simulink model "my_sim"  (R2023b)
settings: Solver=VariableStepAuto  StartTime=0.0  StopTime=2  FixedStep=0.001  MaxStep=0.001  RelTol=1e-3
values from neighbouring files (symbols this model uses):
  Bm = 0.02    [denklemler.m]    (also in my_params.m)
  Freq = 50    [my_params.m]
  J = 0.030    (= 0.03)    [denklemler.m]    (also in my_params.m)
  L1lr = 0.012    [denklemler.m]    (also in my_params.m)
  Lls = 0.008    [denklemler.m]    (also in my_params.m)
  Lm = 0.46    [denklemler.m]    (also in my_params.m)
  P = 2    [denklemler.m]    (also in my_params.m)
  R1r = 1.7    [my_params.m]
  Rs = 2    [denklemler.m]    (also in my_params.m)
  Vampl = 325    [my_params.m]
  w = 2*pi*Freq    (= 314.159265359)    [my_params.m]
libraries: simulink x2, spsabctodq0Lib x1
settings Model: Creator=enesb  LastModifiedBy=enesb
settings DataIOCC: ExternalInput=[inits]  SaveFormat=Array

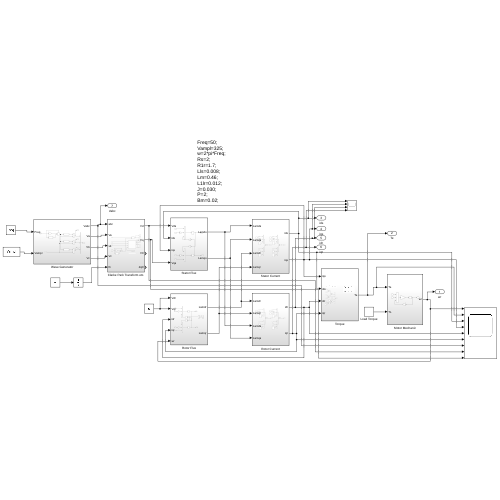
[thumbnail: Simulink's stored preview of the top-level diagram]
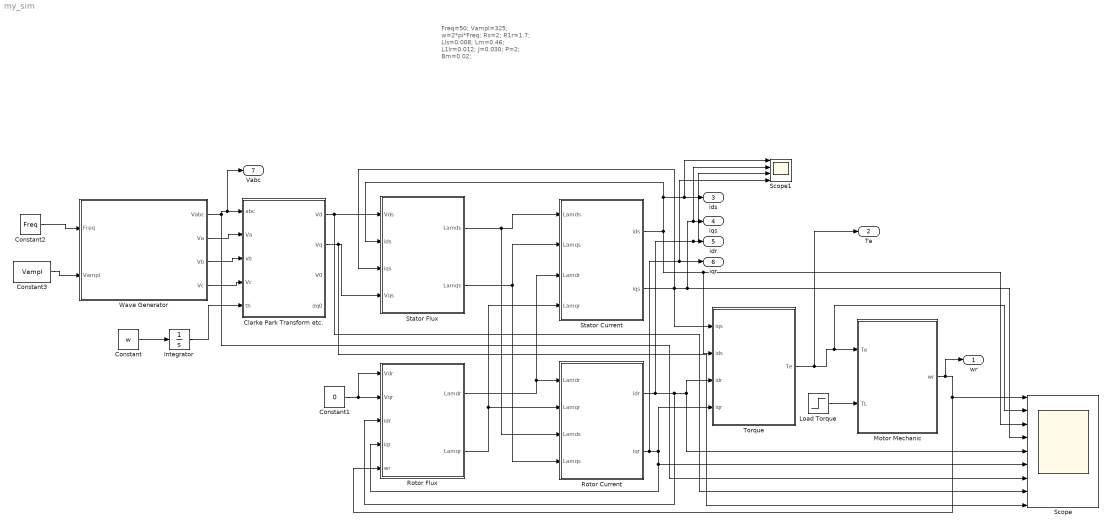
== system my_sim ==
  note: Freq=50;
      | Vampl=325;
      | w=2*pi*Freq;
      | Rs=2;
      | R1r=1.7;
      | Lls=0.008;
      | Lm=0.46;
      | L1lr=0.012;
      | J=0.030;
      | P=2;
      | Bm=0.02;
  Clarke Park Transform etc. : Subsystem
  Constant : Constant  Value=w
  Constant1 : Constant  Value=0
  Constant2 : Constant  Value=Freq
  Constant3 : Constant  Value=Vampl
  Integrator : Integrator
  Load Torque : Step  SampleTime=0
  Motor Mechanic : Subsystem
  Rotor Current : Subsystem
  Rotor Flux : Subsystem
  Scope : Scope  NumInputPorts=9
  Scope1 : Scope  NumInputPorts=4
  Stator Current : Subsystem
  Stator Flux : Subsystem
  Torque : Subsystem
  Wave Generator : Subsystem
  wr : Outport
  Te : Outport  Port=2
  ids : Outport  Port=3
  iqs : Outport  Port=4
  idr : Outport  Port=5
  iqr : Outport  Port=6
  Vabc : Outport  Port=7
  wires:
  Constant2/1 -> Wave Generator/1(Freq)
  Constant3/1 -> Wave Generator/2(Vampl)
  Constant/1 -> Integrator/1
  Wave Generator/1(Vabc) -> Vabc/1, Clarke Park Transform etc./1(abc), Scope/7
  Wave Generator/2(Va) -> Clarke Park Transform etc./2(Va)
  Wave Generator/3(Vb) -> Clarke Park Transform etc./3(vb)
  Wave Generator/4(Vc) -> Clarke Park Transform etc./4(Vc)
  Integrator/1 -> Clarke Park Transform etc./5(th)
  Clarke Park Transform etc./1(Vd) -> Scope/8, Stator Flux/1(Vds)
  Stator Current/1(ids) -> Scope/3, Torque/2(ids), Scope1/1, ids/1, Stator Flux/2(ids)
  Stator Flux/1(Lamds) -> Rotor Current/3(Lamds), Stator Current/1(Lamds)
  Stator Flux/2(Lamqs) -> Stator Current/2(Lamqs), Rotor Current/4(Lamqs)
  Rotor Flux/1(Lamdr) -> Rotor Current/1(Lamdr), Stator Current/3(Lamdr)
  Rotor Flux/2(Lamqr) -> Rotor Current/2(Lamqr), Stator Current/4(Lamqr)
  Clarke Park Transform etc./2(Vq) -> Scope/9, Stator Flux/4(Vqs)
  Rotor Current/1(idr) -> Scope1/3, idr/1, Scope/5, Torque/3(idr), Rotor Flux/3(idr)
  Rotor Current/2(iqr) -> iqr/1, Scope1/4, Torque/4(iqr), Scope/6, Rotor Flux/4(iqr)
  Motor Mechanic/1(wr) -> wr/1, Rotor Flux/5(wr), Scope/1
  Torque/1(Te) -> Te/1, Scope/2, Motor Mechanic/1(Te)
  Load Torque/1 -> Motor Mechanic/2(TL)
  Constant1/1 -> Rotor Flux/1(Vdr), Rotor Flux/2(Vqr)
  Stator Current/2(iqs) -> Scope1/2, iqs/1, Scope/4, Torque/1(iqs), Stator Flux/3(iqs)

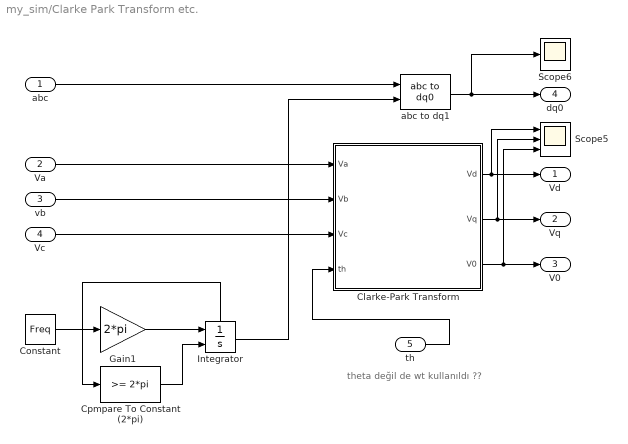
== system my_sim/Clarke Park Transform etc. ==
  note: theta değil de wt kullanıldı ??
  abc : Inport
  Va : Inport  Port=2
  vb : Inport  Port=3
  Vc : Inport  Port=4
  th : Inport  Port=5
  Clarke-Park Transform : MATLAB Function  TreatAsAtomicUnit=on
  Constant : Constant  Value=Freq
  Cpmpare To Constant (2*pi) : simulink/Logic and Bit Operations/Compare To Constant  relop=>=  const=2*pi  OutDataTypeStr=boolean
  Gain1 : Gain  Gain=2*pi
  Integrator : Integrator  ExternalReset=rising  ShowStatePort=on
  Scope5 : Scope  NumInputPorts=3
  Scope6 : Scope
  abc to dq1 : spsabctodq0Lib/abc to dq0  Alignment=90 degrees behind phase A axis
  Vd : Outport
  Vq : Outport  Port=2
  V0 : Outport  Port=3
  dq0 : Outport  Port=4
  wires:
  Vc/1 -> Clarke-Park Transform/3(Vc)
  vb/1 -> Clarke-Park Transform/2(Vb)
  Va/1 -> Clarke-Park Transform/1(Va)
  abc/1 -> abc to dq1/1
  Integrator/1 -> abc to dq1/2
  abc to dq1/1 -> Scope6/1, dq0/1
  Constant/1 -> Gain1/1
  Gain1/1 -> Integrator/1
  Cpmpare To Constant (2*pi)/1 -> Integrator/2
  Integrator/State -> Cpmpare To Constant (2*pi)/1
  Clarke-Park Transform/1(Vd) -> Scope5/1, Vd/1
  Clarke-Park Transform/2(Vq) -> Scope5/2, Vq/1
  Clarke-Park Transform/3(V0) -> Scope5/3, V0/1
  th/1 -> Clarke-Park Transform/4(th)

== system my_sim/Motor Mechanic ==
  Te : Inport
  TL : Inport  Port=2
  Add : Sum  Inputs=+--
  Gain : Gain  Gain=P/(2*J)
  Gain1 : Gain  Gain=Bm
  Integrator1 : Integrator
  wr : Outport
  wires:
  Add/1 -> Gain/1
  TL/1 -> Add/2
  Gain1/1 -> Add/3
  Gain/1 -> Integrator1/1
  Te/1 -> Add/1
  Integrator1/1 -> wr/1, Gain1/1

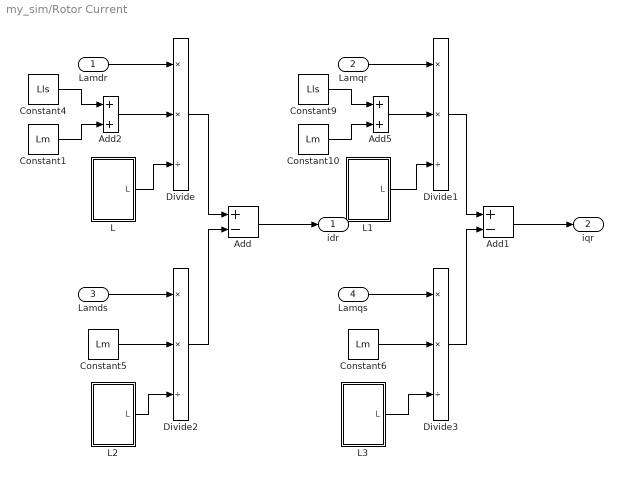
== system my_sim/Rotor Current ==
  Lamdr : Inport
  Lamqr : Inport  Port=2
  Lamds : Inport  Port=3
  Lamqs : Inport  Port=4
  Add : Sum  Inputs=+-
  Add1 : Sum  Inputs=+-
  Add2 : Sum
  Add5 : Sum
  Constant{1,5..6,10} (4 alike) : Constant  Value=Lm
  Constant4 : Constant  Value=Lls
  Constant9 : Constant  Value=Lls
  Divide{,1..3} (4 alike) : Product  Inputs=**/
  L : Subsystem
  L1 : Subsystem
  L2 : Subsystem
  L3 : Subsystem
  idr : Outport
  iqr : Outport  Port=2
  wires:
  Constant4/1 -> Add2/1
  L2/1(L) -> Divide2/3
  L3/1(L) -> Divide3/3
  Add2/1 -> Divide/2
  Constant9/1 -> Add5/1
  Constant1/1 -> Add2/2
  Divide1/1 -> Add1/1
  L1/1(L) -> Divide1/3
  Lamds/1 -> Divide2/1
  Divide3/1 -> Add1/2
  Constant10/1 -> Add5/2
  Add5/1 -> Divide1/2
  L/1(L) -> Divide/3
  Lamdr/1 -> Divide/1
  Constant5/1 -> Divide2/2
  Divide/1 -> Add/1
  Lamqr/1 -> Divide1/1
  Constant6/1 -> Divide3/2
  Lamqs/1 -> Divide3/1
  Add/1 -> idr/1
  Add1/1 -> iqr/1
  Divide2/1 -> Add/2

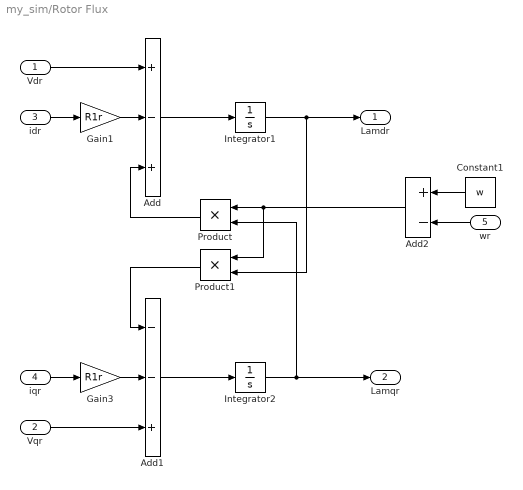
== system my_sim/Rotor Flux ==
  Vdr : Inport
  Vqr : Inport  Port=2
  idr : Inport  Port=3
  iqr : Inport  Port=4
  wr : Inport  Port=5
  Add : Sum  Inputs=+-+
  Add1 : Sum  Inputs=--+
  Add2 : Sum  Inputs=+-
  Constant1 : Constant  Value=w
  Gain1 : Gain  Gain=R1r
  Gain3 : Gain  Gain=R1r
  Integrator1 : Integrator
  Integrator2 : Integrator
  Product : Product
  Product1 : Product
  Lamdr : Outport
  Lamqr : Outport  Port=2
  wires:
  idr/1 -> Gain1/1
  Constant1/1 -> Add2/1
  Product/1 -> Add/3
  Vdr/1 -> Add/1
  Integrator2/1 -> Lamqr/1, Product/2
  iqr/1 -> Gain3/1
  Integrator1/1 -> Lamdr/1, Product1/2
  Gain1/1 -> Add/2
  Vqr/1 -> Add1/3
  Gain3/1 -> Add1/2
  Add/1 -> Integrator1/1
  Add1/1 -> Integrator2/1
  Product1/1 -> Add1/1
  Add2/1 -> Product1/1, Product/1
  wr/1 -> Add2/2

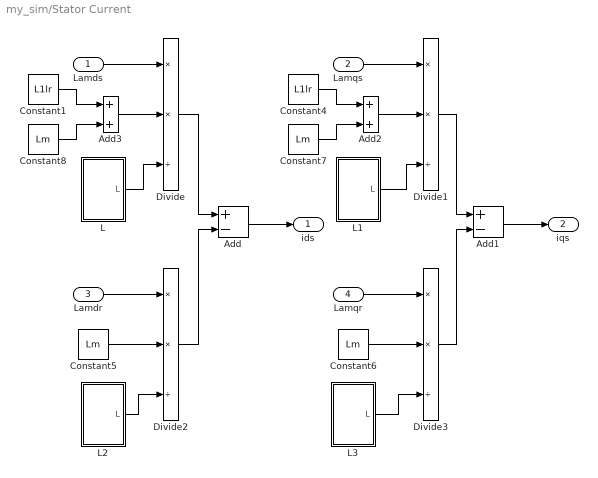
== system my_sim/Stator Current ==
  Lamds : Inport
  Lamqs : Inport  Port=2
  Lamdr : Inport  Port=3
  Lamqr : Inport  Port=4
  Add : Sum  Inputs=+-
  Add1 : Sum  Inputs=+-
  Add2 : Sum
  Add3 : Sum
  Constant1 : Constant  Value=L1lr
  Constant4 : Constant  Value=L1lr
  Constant{5..8} (4 alike) : Constant  Value=Lm
  Divide{,1..3} (4 alike) : Product  Inputs=**/
  L : Subsystem
  L1 : Subsystem
  L2 : Subsystem
  L3 : Subsystem
  ids : Outport
  iqs : Outport  Port=2
  wires:
  Lamqs/1 -> Divide1/1
  Add1/1 -> iqs/1
  Add3/1 -> Divide/2
  L1/1(L) -> Divide1/3
  Add2/1 -> Divide1/2
  Lamqr/1 -> Divide3/1
  Constant5/1 -> Divide2/2
  Lamds/1 -> Divide/1
  Divide1/1 -> Add1/1
  L/1(L) -> Divide/3
  Constant6/1 -> Divide3/2
  Constant8/1 -> Add3/2
  Constant7/1 -> Add2/2
  Constant4/1 -> Add2/1
  L3/1(L) -> Divide3/3
  Constant1/1 -> Add3/1
  Divide2/1 -> Add/2
  Divide/1 -> Add/1
  Lamdr/1 -> Divide2/1
  Divide3/1 -> Add1/2
  Add/1 -> ids/1
  L2/1(L) -> Divide2/3

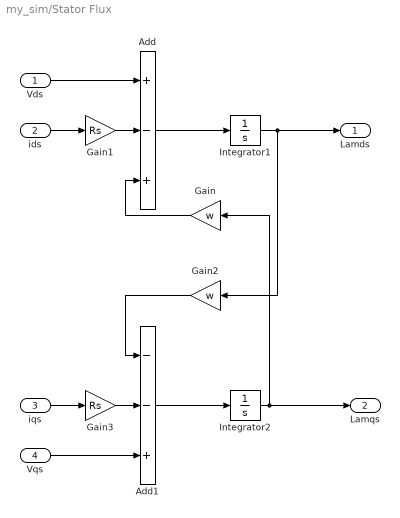
== system my_sim/Stator Flux ==
  Vds : Inport
  ids : Inport  Port=2
  iqs : Inport  Port=3
  Vqs : Inport  Port=4
  Add : Sum  Inputs=+-+
  Add1 : Sum  Inputs=--+
  Gain : Gain  Gain=w
  Gain1 : Gain  Gain=Rs
  Gain2 : Gain  Gain=w
  Gain3 : Gain  Gain=Rs
  Integrator1 : Integrator
  Integrator2 : Integrator
  Lamds : Outport
  Lamqs : Outport  Port=2
  wires:
  Gain1/1 -> Add/2
  ids/1 -> Gain1/1
  Vqs/1 -> Add1/3
  iqs/1 -> Gain3/1
  Gain2/1 -> Add1/1
  Gain/1 -> Add/3
  Vds/1 -> Add/1
  Gain3/1 -> Add1/2
  Integrator2/1 -> Lamqs/1, Gain/1
  Add/1 -> Integrator1/1
  Add1/1 -> Integrator2/1
  Integrator1/1 -> Lamds/1, Gain2/1

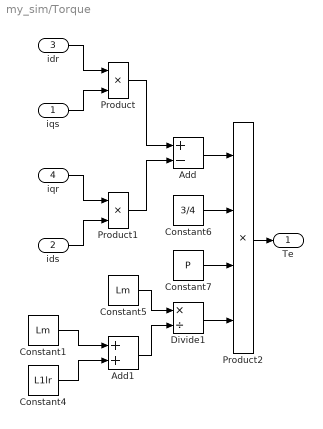
== system my_sim/Torque ==
  iqs : Inport
  ids : Inport  Port=2
  idr : Inport  Port=3
  iqr : Inport  Port=4
  Add : Sum  Inputs=+-
  Add1 : Sum
  Constant1 : Constant  Value=Lm
  Constant4 : Constant  Value=L1lr
  Constant5 : Constant  Value=Lm
  Constant6 : Constant  Value=3/4
  Constant7 : Constant  Value=P
  Divide1 : Product  Inputs=*/
  Product : Product
  Product1 : Product
  Product2 : Product  Inputs=4
  Te : Outport
  wires:
  iqr/1 -> Product1/1
  idr/1 -> Product/1
  Constant6/1 -> Product2/2
  Constant7/1 -> Product2/3
  Constant5/1 -> Divide1/1
  Add1/1 -> Divide1/2
  Product/1 -> Add/1
  Product1/1 -> Add/2
  Constant1/1 -> Add1/1
  iqs/1 -> Product/2
  Product2/1 -> Te/1
  ids/1 -> Product1/2
  Divide1/1 -> Product2/4
  Constant4/1 -> Add1/2
  Add/1 -> Product2/1

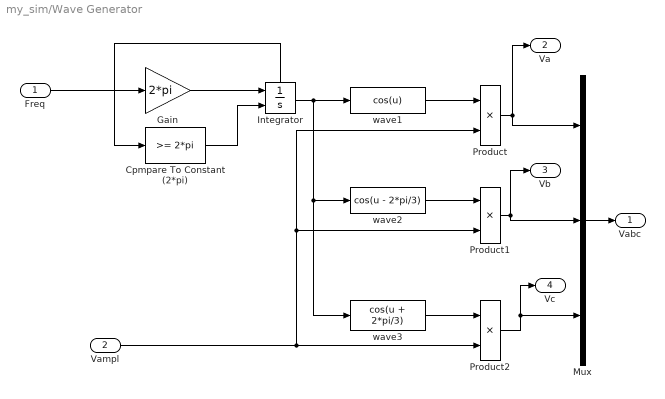
== system my_sim/Wave Generator ==
  Freq : Inport
  Vampl : Inport  Port=2
  Cpmpare To Constant (2*pi) : simulink/Logic and Bit Operations/Compare To Constant  relop=>=  const=2*pi  OutDataTypeStr=boolean
  Gain : Gain  Gain=2*pi
  Integrator : Integrator  ExternalReset=rising  ShowStatePort=on
  Mux : Mux  Inputs=3
  Product : Product
  Product1 : Product
  Product2 : Product
  wave1 : Fcn  Expr=cos(u)
  wave2 : Fcn  Expr=cos(u - 2*pi/3)
  wave3 : Fcn  Expr=cos(u + 2*pi/3)
  Vabc : Outport
  Va : Outport  Port=2
  Vb : Outport  Port=3
  Vc : Outport  Port=4
  wires:
  wave3/1 -> Product2/1
  Product/1 -> Va/1, Mux/1
  wave2/1 -> Product1/1
  Integrator/State -> Cpmpare To Constant (2*pi)/1
  Mux/1 -> Vabc/1
  Gain/1 -> Integrator/1
  Vampl/1 -> Product/2, Product1/2, Product2/2
  wave1/1 -> Product/1
  Cpmpare To Constant (2*pi)/1 -> Integrator/2
  Integrator/1 -> wave1/1, wave3/1, wave2/1
  Product2/1 -> Vc/1, Mux/3
  Product1/1 -> Vb/1, Mux/2
  Freq/1 -> Gain/1

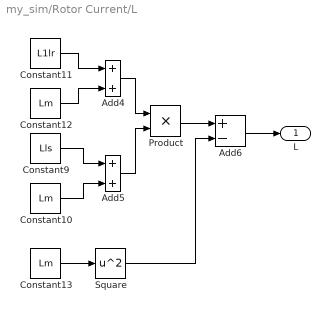
== system my_sim/Rotor Current/L ==
  Add4 : Sum
  Add5 : Sum
  Add6 : Sum  Inputs=+-
  Constant10 : Constant  Value=Lm
  Constant11 : Constant  Value=L1lr
  Constant12 : Constant  Value=Lm
  Constant13 : Constant  Value=Lm
  Constant9 : Constant  Value=Lls
  Product : Product
  Square : Math  Operator=square
  L : Outport
  wires:
  Product/1 -> Add6/1
  Constant12/1 -> Add4/2
  Constant10/1 -> Add5/2
  Add4/1 -> Product/1
  Constant11/1 -> Add4/1
  Constant9/1 -> Add5/1
  Add6/1 -> L/1
  Add5/1 -> Product/2
  Constant13/1 -> Square/1
  Square/1 -> Add6/2

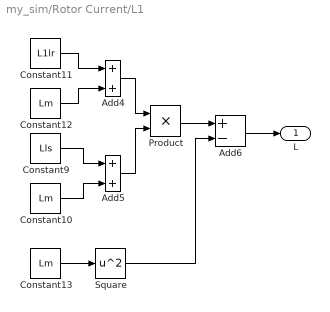
== system my_sim/Rotor Current/L1 ==
  Add4 : Sum
  Add5 : Sum
  Add6 : Sum  Inputs=+-
  Constant10 : Constant  Value=Lm
  Constant11 : Constant  Value=L1lr
  Constant12 : Constant  Value=Lm
  Constant13 : Constant  Value=Lm
  Constant9 : Constant  Value=Lls
  Product : Product
  Square : Math  Operator=square
  L : Outport
  wires:
  Square/1 -> Add6/2
  Constant13/1 -> Square/1
  Add5/1 -> Product/2
  Add6/1 -> L/1
  Constant9/1 -> Add5/1
  Constant11/1 -> Add4/1
  Add4/1 -> Product/1
  Constant10/1 -> Add5/2
  Constant12/1 -> Add4/2
  Product/1 -> Add6/1

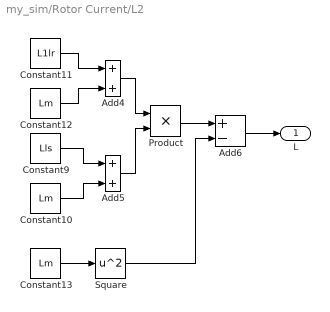
== system my_sim/Rotor Current/L2 ==
  Add4 : Sum
  Add5 : Sum
  Add6 : Sum  Inputs=+-
  Constant10 : Constant  Value=Lm
  Constant11 : Constant  Value=L1lr
  Constant12 : Constant  Value=Lm
  Constant13 : Constant  Value=Lm
  Constant9 : Constant  Value=Lls
  Product : Product
  Square : Math  Operator=square
  L : Outport
  wires:
  Square/1 -> Add6/2
  Constant13/1 -> Square/1
  Add5/1 -> Product/2
  Add6/1 -> L/1
  Constant9/1 -> Add5/1
  Constant11/1 -> Add4/1
  Add4/1 -> Product/1
  Constant10/1 -> Add5/2
  Constant12/1 -> Add4/2
  Product/1 -> Add6/1

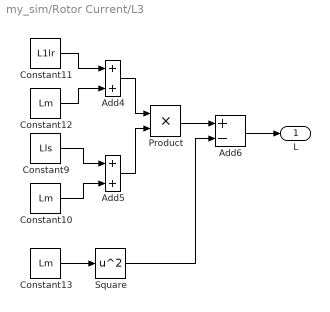
== system my_sim/Rotor Current/L3 ==
  Add4 : Sum
  Add5 : Sum
  Add6 : Sum  Inputs=+-
  Constant10 : Constant  Value=Lm
  Constant11 : Constant  Value=L1lr
  Constant12 : Constant  Value=Lm
  Constant13 : Constant  Value=Lm
  Constant9 : Constant  Value=Lls
  Product : Product
  Square : Math  Operator=square
  L : Outport
  wires:
  Product/1 -> Add6/1
  Constant12/1 -> Add4/2
  Constant10/1 -> Add5/2
  Add4/1 -> Product/1
  Constant11/1 -> Add4/1
  Constant9/1 -> Add5/1
  Add6/1 -> L/1
  Add5/1 -> Product/2
  Constant13/1 -> Square/1
  Square/1 -> Add6/2

== system my_sim/Stator Current/L ==
  Add4 : Sum
  Add5 : Sum
  Add6 : Sum  Inputs=+-
  Constant10 : Constant  Value=Lm
  Constant11 : Constant  Value=L1lr
  Constant12 : Constant  Value=Lm
  Constant13 : Constant  Value=Lm
  Constant9 : Constant  Value=Lls
  Product : Product
  Square : Math  Operator=square
  L : Outport
  wires:
  Product/1 -> Add6/1
  Constant12/1 -> Add4/2
  Constant10/1 -> Add5/2
  Add4/1 -> Product/1
  Constant11/1 -> Add4/1
  Constant9/1 -> Add5/1
  Add6/1 -> L/1
  Add5/1 -> Product/2
  Constant13/1 -> Square/1
  Square/1 -> Add6/2

== system my_sim/Stator Current/L1 ==
  Add4 : Sum
  Add5 : Sum
  Add6 : Sum  Inputs=+-
  Constant10 : Constant  Value=Lm
  Constant11 : Constant  Value=L1lr
  Constant12 : Constant  Value=Lm
  Constant13 : Constant  Value=Lm
  Constant9 : Constant  Value=Lls
  Product : Product
  Square : Math  Operator=square
  L : Outport
  wires:
  Square/1 -> Add6/2
  Constant13/1 -> Square/1
  Add5/1 -> Product/2
  Add6/1 -> L/1
  Constant9/1 -> Add5/1
  Constant11/1 -> Add4/1
  Add4/1 -> Product/1
  Constant10/1 -> Add5/2
  Constant12/1 -> Add4/2
  Product/1 -> Add6/1

== system my_sim/Stator Current/L2 ==
  Add4 : Sum
  Add5 : Sum
  Add6 : Sum  Inputs=+-
  Constant10 : Constant  Value=Lm
  Constant11 : Constant  Value=L1lr
  Constant12 : Constant  Value=Lm
  Constant13 : Constant  Value=Lm
  Constant9 : Constant  Value=Lls
  Product : Product
  Square : Math  Operator=square
  L : Outport
  wires:
  Square/1 -> Add6/2
  Constant13/1 -> Square/1
  Add5/1 -> Product/2
  Add6/1 -> L/1
  Constant9/1 -> Add5/1
  Constant11/1 -> Add4/1
  Add4/1 -> Product/1
  Constant10/1 -> Add5/2
  Constant12/1 -> Add4/2
  Product/1 -> Add6/1

== system my_sim/Stator Current/L3 ==
  Add4 : Sum
  Add5 : Sum
  Add6 : Sum  Inputs=+-
  Constant10 : Constant  Value=Lm
  Constant11 : Constant  Value=L1lr
  Constant12 : Constant  Value=Lm
  Constant13 : Constant  Value=Lm
  Constant9 : Constant  Value=Lls
  Product : Product
  Square : Math  Operator=square
  L : Outport
  wires:
  Product/1 -> Add6/1
  Constant12/1 -> Add4/2
  Constant10/1 -> Add5/2
  Add4/1 -> Product/1
  Constant11/1 -> Add4/1
  Constant9/1 -> Add5/1
  Add6/1 -> L/1
  Add5/1 -> Product/2
  Constant13/1 -> Square/1
  Square/1 -> Add6/2

== matlab function my_sim/Clarke Park Transform etc./Clarke-Park Transform ==
  data: Va input; Vd output; Vb input; Vc input; Vq output; V0 output; th input
function [Vd,Vq,V0]   = ClarkePark(Va,Vb,Vc,th)

% B = [sin(th), sin(th - (2*pi/3)), sin(th + (2*pi/3));
%      cos(th), cos(th - (2*pi/3)), cos(th + (2*pi/3));
%      1/2, 1/2, 1/2];

B = [cos(th), cos(th - (2*pi/3)), cos(th + (2*pi/3));
     sin(th), sin(th - (2*pi/3)), sin(th + (2*pi/3));
     1/2, 1/2, 1/2];

C = [Va; Vb; Vc];



Equ=(2/3)*(B*C);

Vd = Equ(1);
Vq = Equ(2);
V0 = Equ(3);
end
